simulink model "simulation"  (R2017b)
settings: Solver=VariableStepAuto  StartTime=0.0  StopTime=10.0  RelTol=1e-3
values from neighbouring files (symbols this model uses):
  A = [As Bs*Ce; zeros(1,10) Ae]    [ISC_controller.m]
  B = [Bs*De; Be]    [ISC_controller.m]
  C = [Cs Ds*Ce]    [ISC_controller.m]
  ISCS_Ad = sysD.A    [ISC_controller.m]    (also in controller1.mat = [1 0 0 0 0 0 0 0 0 0 0 0 ... (144 elements, 12x12)])
  ISCS_Bd = sysD.B    [ISC_controller.m]    (also in controller1.mat = [1.43765274011e-05 -0.0105531954173 -0.0360066958974 -2.1143)
  ISCS_Cd = sysD.C    [ISC_controller.m]    (also in controller1.mat = [8 0 -0.29381693047 2.72097697141 -0.170864055092 0.67045972)
  ISCS_Dd = sysD.D    [ISC_controller.m]    (also in controller1.mat = [0 0])
  ISCS_Tu = [Tu_alpha; Tu_ign]    [ISC_controller.m]    (also in controller1.mat = [2 -25])
  ISCS_Ty = Ty_omega_e    [ISC_controller.m]    (also in controller1.mat = 107.618371753)
  Ki = 8    [ISC_controller.m]
  L = lqr(A',C',B*B',q)'    [ISC_controller.m]
  Ts = 0.001    [ISC_controller.m]
undefined symbols (not defined in the file or in its folder): DiscIntNeverNeededParam, par
libraries: simulink x1
settings Model: Creator=severinebrunner  LastModifiedBy=niklasbastuck

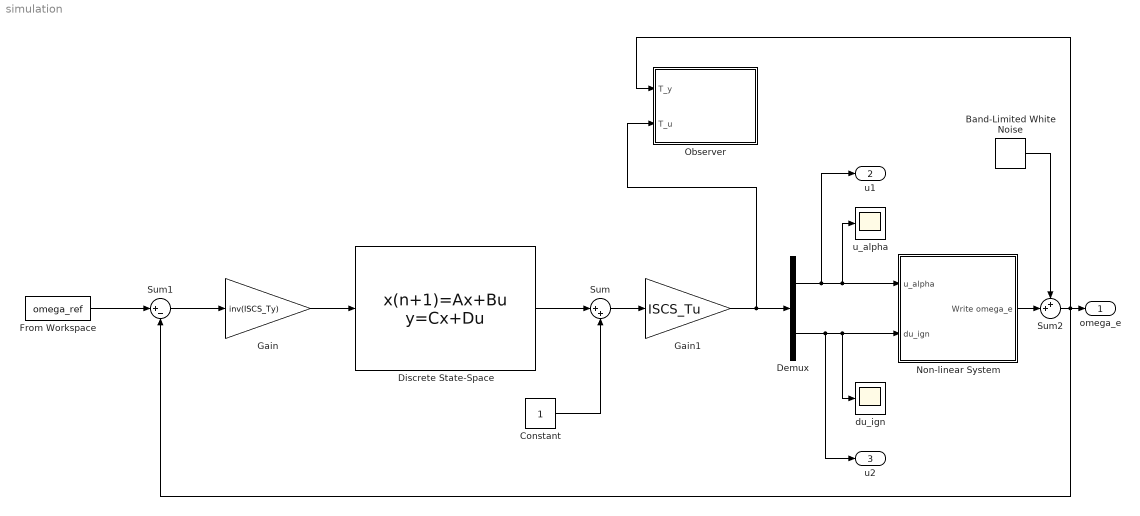
== system simulation ==
  Band-Limited White Noise : simulink/Sources/Band-Limited White Noise  Cov=0.001  Ts=Ts  seed=[23341]
  Constant : Constant
  Demux : Demux  Outputs=2
  Discrete State-Space : DiscreteStateSpace  A=ISCS_Ad  B=ISCS_Bd  C=ISCS_Cd  D=ISCS_Dd  SampleTime=-1
  From Workspace : FromWorkspace  VariableName=omega_ref  SampleTime=0
  Gain : Gain  Gain=inv(ISCS_Ty)
  Gain1 : Gain  Gain=ISCS_Tu
  Non-linear System : Subsystem
  Observer : Subsystem
  Sum : Sum  Inputs=|++
  Sum1 : Sum  Inputs=|+-
  Sum2 : Sum  Inputs=++|
  du_ign : Scope
  u_alpha : Scope
  omega_e : Outport
  u1 : Outport  Port=2
  u2 : Outport  Port=3
  wires:
  Gain/1 -> Discrete State-Space/1
  Discrete State-Space/1 -> Sum/1
  Sum/1 -> Gain1/1
  Constant/1 -> Sum/2
  Demux/1 -> u1/1, Non-linear System/1(u_alpha), u_alpha/1
  Demux/2 -> u2/1, du_ign/1, Non-linear System/2(du_ign)
  Gain1/1 -> Observer/2(T_u), Demux/1
  From Workspace/1 -> Sum1/1
  Sum2/1 -> Sum1/2, Observer/1(T_y), omega_e/1
  Band-Limited White Noise/1 -> Sum2/1
  Non-linear System/1(Write omega_e) -> Sum2/2
  Sum1/1 -> Gain/1

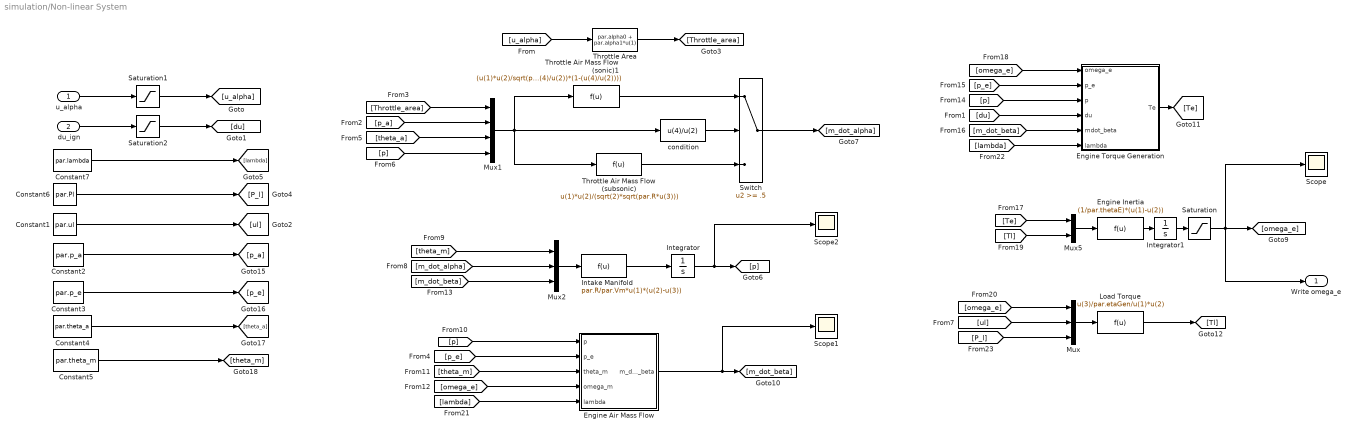
== system simulation/Non-linear System ==
  u_alpha : Inport
  du_ign : Inport  Port=2
  Constant1 : Constant  Value=par.ul
  Constant2 : Constant  Value=par.p_a
  Constant3 : Constant  Value=par.p_e
  Constant4 : Constant  Value=par.theta_a
  Constant5 : Constant  Value=par.theta_m
  Constant6 : Constant  Value=par.Pl
  Constant7 : Constant  Value=par.lambda
  Engine Air Mass Flow : Subsystem
  Engine Inertia : Fcn  Expr=(1/par.thetaE)*(u(1)-u(2))
  Engine Torque Generation : Subsystem
  Intake Manifold : Fcn  Expr=par.R/par.Vm*u(1)*(u(2)-u(3))
  Integrator : Integrator  InitialCondition=par.pm_initial
  Integrator1 : Integrator  InitialCondition=par.omegae_initial
  Load Torque : Fcn  Expr=u(3)/par.etaGen/u(1)*u(2)
  Mux : Mux  Inputs=3
  Mux1 : Mux
  Mux2 : Mux  Inputs=3
  Mux5 : Mux  Inputs=2
  Saturation : Saturate  UpperLimit=500  LowerLimit=20
  Saturation1 : Saturate  UpperLimit=5  LowerLimit=0
  Saturation2 : Saturate  UpperLimit=0  LowerLimit=-100
  Scope : Scope
  Scope1 : Scope
  Scope2 : Scope
  Switch : Switch  Threshold=.5
  Throttle Air Mass Flow (sonic)1 : Fcn  Expr=(u(1)*u(2)/sqrt(par.R*u(3)))*sqrt(2*(u(4)/u(2))*(1-(u(4)/u(2))))
  Throttle Air Mass Flow (subsonic) : Fcn  Expr=u(1)*u(2)/(sqrt(2)*sqrt(par.R*u(3)))
  Throttle Area : Fcn  Expr=par.alpha0 + par.alpha1*u(1)
  "condition " : Fcn  Expr=u(4)/u(2)
  Write omega_e : Outport
  wires:
  Constant3/1 -> [p_e]
  Load Torque/1 -> [Tl]
  Constant5/1 -> [theta_m]
  Engine Air Mass Flow/1(m_dot_beta) -> Scope1/1, [m_dot_beta]
  [theta_a] -> Mux1/3
  Saturation/1 -> Write omega_e/1, Scope/1, [omega_e]
  [lambda] -> Engine Torque Generation/6(lambda)
  [p] -> Mux1/4
  Throttle Area/1 -> [Throttle_area]
  [p_a] -> Mux1/2
  Mux1/1 -> Throttle Air Mass Flow (sonic)1/1, Throttle Air Mass Flow (subsonic)/1, "condition "/1
  [Te] -> Mux5/1
  [theta_m] -> Engine Air Mass Flow/3(theta_m)
  Throttle Air Mass Flow (sonic)1/1 -> Switch/1
  [P_l] -> Mux/3
  [m_dot_alpha] -> Mux2/2
  Constant4/1 -> [theta_a]
  Throttle Air Mass Flow (subsonic)/1 -> Switch/3
  [p_e] -> Engine Air Mass Flow/2(p_e)
  [m_dot_beta] -> Mux2/3
  "condition "/1 -> Switch/2
  Intake Manifold/1 -> Integrator/1
  [lambda] -> Engine Air Mass Flow/5(lambda)
  [Throttle_area] -> Mux1/1
  [p_e] -> Engine Torque Generation/2(p_e)
  Constant1/1 -> [ul]
  Engine Torque Generation/1("Te ") -> [Te]
  [omega_e] -> Engine Torque Generation/1(omega_e)
  [omega_e] -> Mux/1
  [ul] -> Mux/2
  [u_alpha] -> Throttle Area/1
  [p] -> Engine Air Mass Flow/1(p)
  Integrator/1 -> Scope2/1, [p]
  [omega_e] -> Engine Air Mass Flow/4(omega_m)
  Constant6/1 -> [P_l]
  Mux5/1 -> Engine Inertia/1
  Constant2/1 -> [p_a]
  [p] -> Engine Torque Generation/3(p)
  Constant7/1 -> [lambda]
  [m_dot_beta] -> Engine Torque Generation/5(mdot_beta)
  [du] -> Engine Torque Generation/4(du)
  Engine Inertia/1 -> Integrator1/1
  [theta_m] -> Mux2/1
  Mux/1 -> Load Torque/1
  Integrator1/1 -> Saturation/1
  Mux2/1 -> Intake Manifold/1
  Switch/1 -> [m_dot_alpha]
  [Tl] -> Mux5/2
  u_alpha/1 -> Saturation1/1
  Saturation1/1 -> [u_alpha]
  Saturation2/1 -> [du]
  du_ign/1 -> Saturation2/1

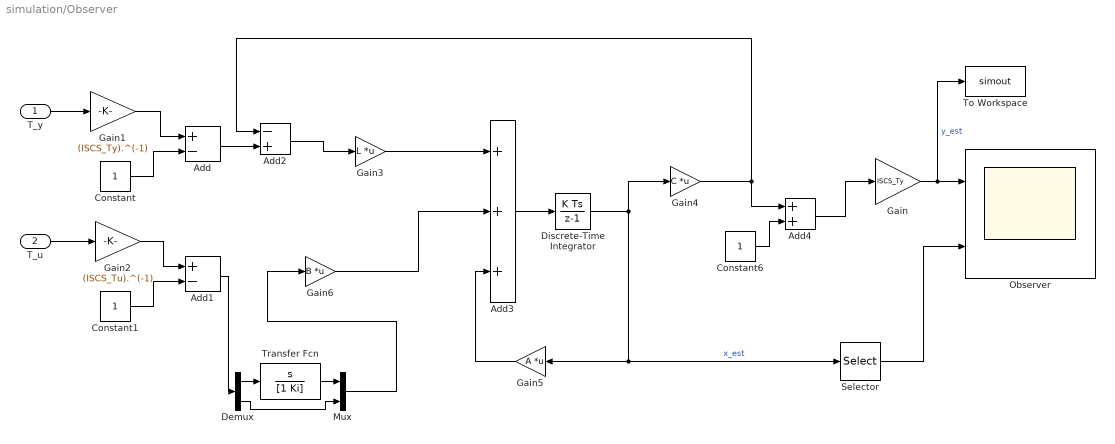
== system simulation/Observer ==
  T_y : Inport
  T_u : Inport  Port=2
  Add : Sum  Inputs=+-
  Add1 : Sum  Inputs=+-
  Add2 : Sum  Inputs=-+
  Add3 : Sum  Inputs=+++
  Add4 : Sum
  Constant : Constant
  Constant1 : Constant
  Constant6 : Constant
  Demux : Demux  Outputs=2
  Discrete-Time Integrator : DiscreteIntegrator  InitialCondition=[(par.omegae_initial-ISCS_Ty)/ISCS_Ty zeros(1,10) ]  InitialConditionSetting=State (most efficient)  SampleTime=Ts  ICPrevOutput=DiscIntNeverNeededParam  ICPrevScaledInput=DiscIntNeverNeededParam
  Gain : Gain  Gain=ISCS_Ty
  Gain1 : Gain  Gain=(ISCS_Ty).^(-1)
  Gain2 : Gain  Gain=(ISCS_Tu).^(-1)
  Gain3 : Gain  Gain=L  Multiplication=Matrix(K*u)
  Gain4 : Gain  Gain=C  Multiplication=Matrix(K*u)
  Gain5 : Gain  Gain=A  Multiplication=Matrix(K*u)
  Gain6 : Gain  Gain=B  Multiplication=Matrix(K*u)
  Mux : Mux  Inputs=2
  Observer : Scope  NumInputPorts=2
  Selector : Selector  InputPortWidth=11  IndexOptions=Index vector (dialog)  Indices=1  OutputSizes=1
  To Workspace : ToWorkspace  VariableName=simout  SaveFormat=Timeseries  SampleTime=-1
  Transfer Fcn : TransferFcn  Numerator=[1 0]  Denominator=[1 Ki]
  wires:
  Constant/1 -> Add/2
  Constant1/1 -> Add1/2
  Gain6/1 -> Add3/2
  Add/1 -> Add2/2
  Gain4/1 -> Add4/1, Add2/1
  Constant6/1 -> Add4/2
  Gain/1 -> To Workspace/1, Observer/1  "y_est"
  Gain2/1 -> Add1/1
  T_u/1 -> Gain2/1
  Add4/1 -> Gain/1
  Selector/1 -> Observer/2
  Discrete-Time Integrator/1 -> Gain4/1, Gain5/1, Selector/1  "x_est"
  T_y/1 -> Gain1/1
  Gain1/1 -> Add/1
  Add3/1 -> Discrete-Time Integrator/1
  Demux/1 -> Transfer Fcn/1
  Transfer Fcn/1 -> Mux/1
  Demux/2 -> Mux/2
  Add1/1 -> Demux/1
  Gain3/1 -> Add3/1
  Add2/1 -> Gain3/1
  Gain5/1 -> Add3/3
  Mux/1 -> Gain6/1

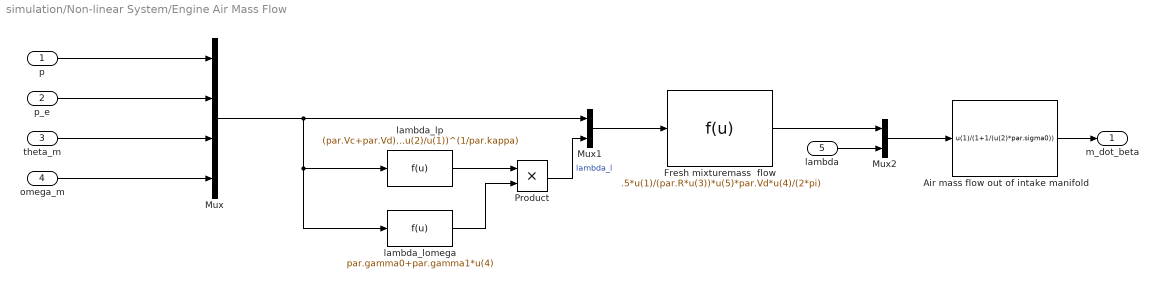
== system simulation/Non-linear System/Engine Air Mass Flow ==
  p : Inport
  p_e : Inport  Port=2
  theta_m : Inport  Port=3
  omega_m : Inport  Port=4
  lambda : Inport  Port=5
  Air mass flow out of intake manifold : Fcn  Expr=u(1)/(1+1/(u(2)*par.sigma0))
  Fresh mixturemass  flow : Fcn  Expr=.5*u(1)/(par.R*u(3))*u(5)*par.Vd*u(4)/(2*pi)
  Mux : Mux
  Mux1 : Mux  Inputs=2
  Mux2 : Mux  Inputs=2
  Product : Product
  lambda_lomega : Fcn  Expr=par.gamma0+par.gamma1*u(4)
  lambda_lp : Fcn  Expr=(par.Vc+par.Vd)/par.Vd - (par.Vc/par.Vd)*(u(2)/u(1))^(1/par.kappa)
  m_dot_beta : Outport
  wires:
  p/1 -> Mux/1
  p_e/1 -> Mux/2
  theta_m/1 -> Mux/3
  omega_m/1 -> Mux/4
  Mux/1 -> lambda_lomega/1, lambda_lp/1, Mux1/1
  lambda_lp/1 -> Product/1
  lambda_lomega/1 -> Product/2
  Product/1 -> Mux1/2  "lambda_l"
  Mux1/1 -> Fresh mixturemass  flow/1
  Fresh mixturemass  flow/1 -> Mux2/1
  Air mass flow out of intake manifold/1 -> m_dot_beta/1
  lambda/1 -> Mux2/2
  Mux2/1 -> Air mass flow out of intake manifold/1

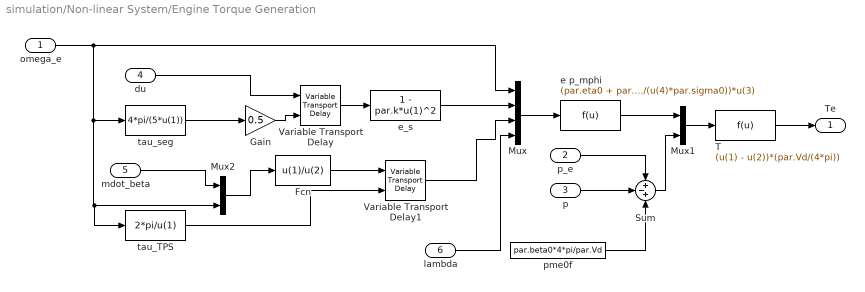
== system simulation/Non-linear System/Engine Torque Generation ==
  omega_e : Inport
  p_e : Inport  Port=2
  p : Inport  Port=3
  du : Inport  Port=4
  mdot_beta : Inport  Port=5
  lambda : Inport  Port=6
  Fcn : Fcn  Expr=u(1)/u(2)
  Gain : Gain  Gain=0.5
  Mux : Mux
  Mux1 : Mux  Inputs=2
  Mux2 : Mux  Inputs=2
  Sum : Sum  Inputs=+-+
  T : Fcn  Expr=(u(1) - u(2))*(par.Vd/(4*pi))
  Variable Transport Delay : VariableTransportDelay  MaximumDelay=10  InitialOutput=par.ss_duign  MaximumPoints=10240
  Variable Transport Delay1 : VariableTransportDelay  MaximumDelay=10  InitialOutput=par.ss_mdotalpha/par.ss_omegae  MaximumPoints=10240
  e p_mphi : Fcn  Expr=(par.eta0 + par.eta1*u(1))*u(2)*(par.Hl/par.Vd)*(4*pi/(u(4)*par.sigma0))*u(3)
  e_s : Fcn  Expr=1 - par.k*u(1)^2
  pme0f : Constant  Value=par.beta0*4*pi/par.Vd  VectorParams1D=off
  tau_TPS : Fcn  Expr=2*pi/u(1)
  tau_seg : Fcn  Expr=4*pi/(5*u(1))
  "Te " : Outport
  wires:
  du/1 -> Variable Transport Delay/1
  tau_seg/1 -> Gain/1
  Mux1/1 -> T/1
  omega_e/1 -> Mux2/2, tau_TPS/1, tau_seg/1, Mux/1
  Variable Transport Delay1/1 -> Mux/3
  mdot_beta/1 -> Mux2/1
  tau_TPS/1 -> Variable Transport Delay1/2
  p/1 -> Sum/2
  Gain/1 -> Variable Transport Delay/2
  p_e/1 -> Sum/1
  Sum/1 -> Mux1/2
  Mux/1 -> e p_mphi/1
  e_s/1 -> Mux/2
  e p_mphi/1 -> Mux1/1
  Variable Transport Delay/1 -> e_s/1
  T/1 -> "Te "/1
  Mux2/1 -> Fcn/1
  Fcn/1 -> Variable Transport Delay1/1
  lambda/1 -> Mux/4
  pme0f/1 -> Sum/3
